simulink model "DTSMC_Gao_TWMR_Position"  (R2018b)
settings: Solver=FixedStepAuto  StartTime=0.0  StopTime=100  FixedStep=0.01  RelTol=1e-3
values from neighbouring files (symbols this model uses):
  c = K'    [DTSMC_Gao_TWMR_Position_param.m]    (also in DTSMC_Gao_TWMR_velocity_param.m; robotprojectvalues.m = 0.5)
  c1 = c(1)    [DTSMC_Gao_TWMR_Position_param.m]    (also in DTSMC_Gao_TWMR_velocity_param.m)
  c2 = c(2)    [DTSMC_Gao_TWMR_Position_param.m]    (also in DTSMC_Gao_TWMR_velocity_param.m = 0)
  Gam_tau = [5e-5; 0.01]    [DTSMC_Gao_TWMR_Position_param.m]    (also in DTSMC_Gao_TWMR_velocity_param.m = [0;1])
libraries: simulink x1
settings Model: Creator=HP  LastModifiedBy=baleshwar
settings SFSimCC: SimUseLocalCustomCode=off
settings RTWCC: RTWUseLocalCustomCode=off
settings CodeAppCC: StateflowObjectComments=on

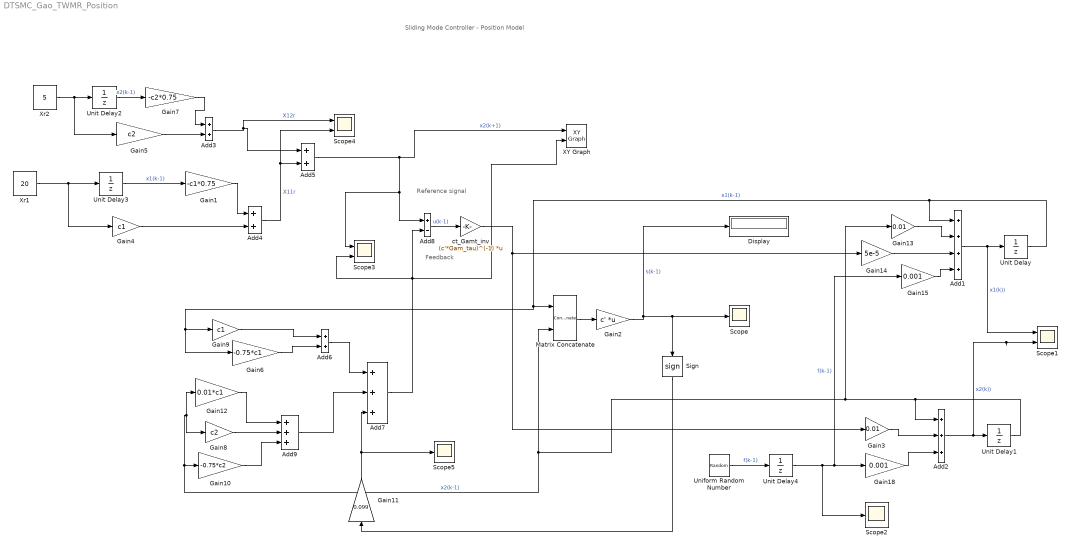
== system DTSMC_Gao_TWMR_Position ==
  note: Sliding Mode Controller - Position Model
  note: Reference signal
  note: Feedback
  Add1 : Sum  Inputs=++++
  Add2 : Sum  Inputs=+++
  Add{3..6} (4 alike) : Sum
  Add7 : Sum  Inputs=+++
  Add8 : Sum  Inputs=+-
  Add9 : Sum  Inputs=+++
  Display : Display
  Gain1 : Gain  Gain=-c1*0.75
  Gain10 : Gain  Gain=-0.75*c2
  Gain11 : Gain  Gain=0.099
  Gain12 : Gain  Gain=0.01*c1
  Gain13 : Gain  Gain=0.01
  Gain14 : Gain  Gain=5e-5
  Gain15 : Gain  Gain=0.001
  Gain18 : Gain  Gain=0.001
  Gain2 : Gain  Gain=c'  Multiplication=Matrix(K*u)
  Gain3 : Gain  Gain=0.01
  Gain4 : Gain  Gain=c1
  Gain5 : Gain  Gain=c2
  Gain6 : Gain  Gain=-0.75*c1
  Gain7 : Gain  Gain=-c2*0.75
  Gain8 : Gain  Gain=c2
  Gain9 : Gain  Gain=c1
  Matrix Concatenate : Concatenate  Mode=Multidimensional array
  Scope : Scope
  Scope1 : Scope  NumInputPorts=2
  Scope2 : Scope
  Scope3 : Scope  NumInputPorts=2
  Scope4 : Scope  NumInputPorts=2
  Scope5 : Scope
  Sign : Signum
  Uniform Random Number : UniformRandomNumber  Minimum=-0.05  Maximum=0.05  SampleTime=0.01
  Unit Delay : UnitDelay  SampleTime=0.01
  Unit Delay1 : UnitDelay  SampleTime=0.01
  Unit Delay2 : UnitDelay  SampleTime=0.1
  Unit Delay3 : UnitDelay  SampleTime=0.1
  Unit Delay4 : UnitDelay  SampleTime=0.1
  XY Graph : simulink/Sinks/XY Graph  xmin=-inf  xmax=inf  ymin=-inf  ymax=inf  st=0.1
  Xr1 : Constant  Value=20  SampleTime=0.01
  "Xr2 " : Constant  Value=5  SampleTime=0.01
  ct_Gamt_inv : Gain  Gain=(c'*Gam_tau)^(-1)  Multiplication=Matrix(K*u)
  wires:
  Gain7/1 -> Add3/1
  Unit Delay2/1 -> Gain7/1  "x2(k-1)"
  Gain5/1 -> Add3/2
  Unit Delay3/1 -> Gain1/1  "x1(k-1)"
  Gain4/1 -> Add4/2
  "Xr2 "/1 -> Gain5/1, Unit Delay2/1
  Xr1/1 -> Unit Delay3/1, Gain4/1
  Add4/1 -> Add5/2, Scope4/2  "X11r"
  Gain9/1 -> Add6/1
  Add6/1 -> Add7/1
  Gain2/1 -> Display/1, Scope/1, Sign/1  "s(k-1)"
  Unit Delay/1 -> Add1/1, Matrix Concatenate/1, Gain6/1, Gain9/1  "x1(k-1)"
  Gain13/1 -> Add1/2
  Gain14/1 -> Add1/3
  Gain15/1 -> Add1/4
  Add1/1 -> Scope1/1, Unit Delay/1  "x1(k))"
  Add2/1 -> Scope1/2, Unit Delay1/1  "x2(k))"
  Unit Delay1/1 -> Gain13/1, Matrix Concatenate/2, Gain12/1, Gain8/1, Gain10/1, Add2/1  "x2(k-1)"
  Gain18/1 -> Add2/3
  Gain3/1 -> Add2/2
  Add8/1 -> ct_Gamt_inv/1  "u(k-1)"
  Sign/1 -> Gain11/1
  Uniform Random Number/1 -> Unit Delay4/1  "f(k-1)"
  Add7/1 -> XY Graph/2, Scope3/2, Add8/2
  Unit Delay4/1 -> Scope2/1, Gain18/1, Gain15/1  "f(k-1)"
  Add5/1 -> Scope3/1, Add8/1, XY Graph/1  "x2(k+1)"
  Matrix Concatenate/1 -> Gain2/1
  ct_Gamt_inv/1 -> Gain14/1, Gain3/1
  Gain1/1 -> Add4/1
  Gain6/1 -> Add6/2
  Gain12/1 -> Add9/1
  Gain8/1 -> Add9/2
  Gain10/1 -> Add9/3
  Add9/1 -> Add7/2
  Gain11/1 -> Scope5/1, Add7/3
  Add3/1 -> Add5/1, Scope4/1  "X12r"
